simulink model "Model_TranslationEngine64"  (R2022b)
settings: Solver=FixedStepDiscrete  StartTime=0.0  StopTime=5  RelTol=1e-3  EnableMultiTasking=on
InitFcn:
  | % Initialize model
  | ModelSettings=BTConfig.GetModelSettings();
  | 
  | ModelSettings.Validate();
  | 
  | ModelInit;
  | 
  | 
  | % load library data
  | GainLibrary_data;
  | % Load saved values from partition process
  | CapturedConstMask.LoadMapFromFile(bdroot)
StartFcn:
  | % make sure all the simulated RTC requests are found
  | %RTC_SIM_OBJ.ValidateREQs();
undefined symbols (not defined in the file or in its folder): AA, BPLP, Column, NumHFRefBPF, NumHFRefLPF, NumMusicChannels, Row, VolumeMuteConfig
libraries: TuneVar x925, TOP x490, FeaturePath x111, CapturedConstLib x52
(part 10 of 34)

== system Model_TranslationEngine64/NEAR/Near1p1/VolumeMute/VolMuteCh4/Ann4NonEntGainCalc ==
  FeaturePath : FeaturePath/FeaturePath  FeatureName=Ann4NonEntGainCalc  IsGroup=off  GroupNumber=-1  IsModule=off  TriggerInit=[-350 -126 -235 -19]
      settings: SourceProductName=Bose Talaria
  TuneTOP : Subsystem  mask(Talaria Trivial Tune TOP){TriggerInit=[-380 277 -210 333], TopName=VncThresh, TuneName=VncThresh, DataTypeOut=single, MaskValue=Config.DefaultVncThresh, TunabilityNumber=1, MinValue=[], MaxValue=[], BankNumber=0, PreOverlay=false, PostOverlay=false, UseSameName=on}
      mask prompts: TriggerInit "Hidden: MoveFcn redraw"; TopName "Name:"; TuneName "Name of TuneVar:"; DataTypeOut "Data type:"; MaskValue "Default Value:"; TunabilityNumber "Tunability:"; MinValue "Min Value:"; MaxValue "Max Value:"; BankNumber "Target memory bank number:"; PreOverlay "Requires pre-overlay action:"; PostOverlay "Requires post-overlay action:"; UseSameName "Use same name for tune variable and TOP"
      mask help: The TuneTOP block encapsultes a Target Overlay Parameter, a Tune Variable, and a Trivial Translation between them.
      mask init:
      | [ok,activeTopPath,activeTunePath] = TuneTOP_Mask.Init(gcbh);
      settings: MoveFcn=TuneTOP_Mask.CB_TriggerInit(gcbh);
      mask Callback TriggerInit: TuneTOP_Mask.CB_TriggerInit(gcbh);
      mask TypeOptions TopName: TOP/TopName
      mask TypeOptions TuneName: Tune Variable/TuneName
      mask TypeOptions DataTypeOut: TOP/DataTypeOut
      mask TypeOptions MaskValue: Tune Variable/MaskValue
      mask TypeOptions TunabilityNumber: Tune Variable/TunabilityNumber
      mask Callback TunabilityNumber: TuneVarMask.CB_TunabilityNumber(gcbh);
      mask TypeOptions MinValue: Tune Variable/MinValue
      mask TypeOptions MaxValue: Tune Variable/MaxValue
      mask TypeOptions BankNumber: TOP/BankNumber
      mask TypeOptions PreOverlay: TOP/PreOverlay
      mask TypeOptions PostOverlay: TOP/PostOverlay
      mask Callback UseSameName: TuneTOP_Mask.CB_UseSameName(gcbh);
      mask DialogControl toolPanel Prompt: Tuning Tool Hints
      mask DialogControl DescriptionGroup Prompt: Description
      mask DialogControl EditDescription Prompt: Edit Description
      mask DialogControl EditDescription Callback: TuneTOP_Mask.CB_EditDescription(gcbh);
      mask DialogControl TunabilityText Prompt: Easy: Changes nearly every tuning.
      mask DialogControl AdvancedPanel Prompt: Advanced
      mask DialogControl ConvertToFullTranslation Prompt: Irreversible conversion to full translation
      mask DialogControl ConvertToFullTranslation Callback: TuneTOP_Mask.CB_ConvertToFullTranslation(gcbh);
      mask DialogControl ErrorContainer Prompt: Error Messages
      mask Display:
      | % retrieve icon definition
      | [path,w,h] = TuneTOP_Mask.Icon();
      | 
      | % retrieve the block's pixel size
      | pos = get(gcbh,'position');
      | bw = pos(3) - pos(1);
      | bh = pos(4) - pos(2);
      | 
      | % draw centered icon
      | xAdj = bw/2 - w/2 + 5;
      | yAdj = bh/2 - h/2 + 4;
      | for i=1:length(path)
      | 	patch(path(i).x+xAdj, path(i).y+yAdj, path(i).rgb);
      | end
      | 
      | % show the top name or an X
      | if (exist('ok','var') && ok)
      | 	text(bw*0.5, bh*0.2, activeTopPath, 'horizontalAlignment', 'center');
      | 	patch(0,0,[1 1 1]);
      | 	patch(bw,bh,[1 1 1]);
      | else
      | 	tx=bw*0.03;
      | 	ty=bh*0.03;
      | 	patch([0 tx bw bw-tx], [ty 0 bh-ty bh], [1 0 0]);
      | 	patch([0 bw-tx bw tx], [bh-ty 0 ty bh], [1 0 0]);
      | end
  TuneTOP1 : Subsystem  mask(Talaria Trivial Tune TOP){TriggerInit=[-380 347 -210 403], TopName=VncSlope, TuneName=VncSlope, DataTypeOut=single, MaskValue=Config.DefaultVncSlope, TunabilityNumber=1, MinValue=[], MaxValue=[], BankNumber=0, PreOverlay=false, PostOverlay=false, UseSameName=on}
      mask prompts: TriggerInit "Hidden: MoveFcn redraw"; TopName "Name:"; TuneName "Name of TuneVar:"; DataTypeOut "Data type:"; MaskValue "Default Value:"; TunabilityNumber "Tunability:"; MinValue "Min Value:"; MaxValue "Max Value:"; BankNumber "Target memory bank number:"; PreOverlay "Requires pre-overlay action:"; PostOverlay "Requires post-overlay action:"; UseSameName "Use same name for tune variable and TOP"
      mask help: The TuneTOP block encapsultes a Target Overlay Parameter, a Tune Variable, and a Trivial Translation between them.
      mask init:
      | [ok,activeTopPath,activeTunePath] = TuneTOP_Mask.Init(gcbh);
      settings: MoveFcn=TuneTOP_Mask.CB_TriggerInit(gcbh);
      mask Callback TriggerInit: TuneTOP_Mask.CB_TriggerInit(gcbh);
      mask TypeOptions TopName: TOP/TopName
      mask TypeOptions TuneName: Tune Variable/TuneName
      mask TypeOptions DataTypeOut: TOP/DataTypeOut
      mask TypeOptions MaskValue: Tune Variable/MaskValue
      mask TypeOptions TunabilityNumber: Tune Variable/TunabilityNumber
      mask Callback TunabilityNumber: TuneVarMask.CB_TunabilityNumber(gcbh);
      mask TypeOptions MinValue: Tune Variable/MinValue
      mask TypeOptions MaxValue: Tune Variable/MaxValue
      mask TypeOptions BankNumber: TOP/BankNumber
      mask TypeOptions PreOverlay: TOP/PreOverlay
      mask TypeOptions PostOverlay: TOP/PostOverlay
      mask Callback UseSameName: TuneTOP_Mask.CB_UseSameName(gcbh);
      mask DialogControl toolPanel Prompt: Tuning Tool Hints
      mask DialogControl DescriptionGroup Prompt: Description
      mask DialogControl EditDescription Prompt: Edit Description
      mask DialogControl EditDescription Callback: TuneTOP_Mask.CB_EditDescription(gcbh);
      mask DialogControl TunabilityText Prompt: Easy: Changes nearly every tuning.
      mask DialogControl AdvancedPanel Prompt: Advanced
      mask DialogControl ConvertToFullTranslation Prompt: Irreversible conversion to full translation
      mask DialogControl ConvertToFullTranslation Callback: TuneTOP_Mask.CB_ConvertToFullTranslation(gcbh);
      mask DialogControl ErrorContainer Prompt: Error Messages
      mask Display:
      | % retrieve icon definition
      | [path,w,h] = TuneTOP_Mask.Icon();
      | 
      | % retrieve the block's pixel size
      | pos = get(gcbh,'position');
      | bw = pos(3) - pos(1);
      | bh = pos(4) - pos(2);
      | 
      | % draw centered icon
      | xAdj = bw/2 - w/2 + 5;
      | yAdj = bh/2 - h/2 + 4;
      | for i=1:length(path)
      | 	patch(path(i).x+xAdj, path(i).y+yAdj, path(i).rgb);
      | end
      | 
      | % show the top name or an X
      | if (exist('ok','var') && ok)
      | 	text(bw*0.5, bh*0.2, activeTopPath, 'horizontalAlignment', 'center');
      | 	patch(0,0,[1 1 1]);
      | 	patch(bw,bh,[1 1 1]);
      | else
      | 	tx=bw*0.03;
      | 	ty=bh*0.03;
      | 	patch([0 tx bw bw-tx], [ty 0 bh-ty bh], [1 0 0]);
      | 	patch([0 bw-tx bw tx], [bh-ty 0 ty bh], [1 0 0]);
      | end
  TuneTOP2 : Subsystem  mask(Talaria Trivial Tune TOP){TriggerInit=[-380 427 -210 483], TopName=MaxBoost, TuneName=MaxBoost, DataTypeOut=single, MaskValue=Config.DefaultMaxBoost, TunabilityNumber=1, MinValue=[], MaxValue=[], BankNumber=0, PreOverlay=false, PostOverlay=false, UseSameName=on}
      mask prompts: TriggerInit "Hidden: MoveFcn redraw"; TopName "Name:"; TuneName "Name of TuneVar:"; DataTypeOut "Data type:"; MaskValue "Default Value:"; TunabilityNumber "Tunability:"; MinValue "Min Value:"; MaxValue "Max Value:"; BankNumber "Target memory bank number:"; PreOverlay "Requires pre-overlay action:"; PostOverlay "Requires post-overlay action:"; UseSameName "Use same name for tune variable and TOP"
      mask help: The TuneTOP block encapsultes a Target Overlay Parameter, a Tune Variable, and a Trivial Translation between them.
      mask init:
      | [ok,activeTopPath,activeTunePath] = TuneTOP_Mask.Init(gcbh);
      settings: MoveFcn=TuneTOP_Mask.CB_TriggerInit(gcbh);
      mask Callback TriggerInit: TuneTOP_Mask.CB_TriggerInit(gcbh);
      mask TypeOptions TopName: TOP/TopName
      mask TypeOptions TuneName: Tune Variable/TuneName
      mask TypeOptions DataTypeOut: TOP/DataTypeOut
      mask TypeOptions MaskValue: Tune Variable/MaskValue
      mask TypeOptions TunabilityNumber: Tune Variable/TunabilityNumber
      mask Callback TunabilityNumber: TuneVarMask.CB_TunabilityNumber(gcbh);
      mask TypeOptions MinValue: Tune Variable/MinValue
      mask TypeOptions MaxValue: Tune Variable/MaxValue
      mask TypeOptions BankNumber: TOP/BankNumber
      mask TypeOptions PreOverlay: TOP/PreOverlay
      mask TypeOptions PostOverlay: TOP/PostOverlay
      mask Callback UseSameName: TuneTOP_Mask.CB_UseSameName(gcbh);
      mask DialogControl toolPanel Prompt: Tuning Tool Hints
      mask DialogControl DescriptionGroup Prompt: Description
      mask DialogControl EditDescription Prompt: Edit Description
      mask DialogControl EditDescription Callback: TuneTOP_Mask.CB_EditDescription(gcbh);
      mask DialogControl TunabilityText Prompt: Easy: Changes nearly every tuning.
      mask DialogControl AdvancedPanel Prompt: Advanced
      mask DialogControl ConvertToFullTranslation Prompt: Irreversible conversion to full translation
      mask DialogControl ConvertToFullTranslation Callback: TuneTOP_Mask.CB_ConvertToFullTranslation(gcbh);
      mask DialogControl ErrorContainer Prompt: Error Messages
      mask Display:
      | % retrieve icon definition
      | [path,w,h] = TuneTOP_Mask.Icon();
      | 
      | % retrieve the block's pixel size
      | pos = get(gcbh,'position');
      | bw = pos(3) - pos(1);
      | bh = pos(4) - pos(2);
      | 
      | % draw centered icon
      | xAdj = bw/2 - w/2 + 5;
      | yAdj = bh/2 - h/2 + 4;
      | for i=1:length(path)
      | 	patch(path(i).x+xAdj, path(i).y+yAdj, path(i).rgb);
      | end
      | 
      | % show the top name or an X
      | if (exist('ok','var') && ok)
      | 	text(bw*0.5, bh*0.2, activeTopPath, 'horizontalAlignment', 'center');
      | 	patch(0,0,[1 1 1]);
      | 	patch(bw,bh,[1 1 1]);
      | else
      | 	tx=bw*0.03;
      | 	ty=bh*0.03;
      | 	patch([0 tx bw bw-tx], [ty 0 bh-ty bh], [1 0 0]);
      | 	patch([0 bw-tx bw tx], [bh-ty 0 ty bh], [1 0 0]);
      | end
  TuneTOP3 : Subsystem  mask(Talaria Trivial Tune TOP){TriggerInit=[-760 -98 -590 -42], TopName=NoiseOverRide, TuneName=NoiseOverRide, DataTypeOut=single, MaskValue=Config.DefaultNoiseOverride, TunabilityNumber=1, MinValue=[], MaxValue=[], BankNumber=0, PreOverlay=false, PostOverlay=false, UseSameName=on}
      mask prompts: TriggerInit "Hidden: MoveFcn redraw"; TopName "Name:"; TuneName "Name of TuneVar:"; DataTypeOut "Data type:"; MaskValue "Default Value:"; TunabilityNumber "Tunability:"; MinValue "Min Value:"; MaxValue "Max Value:"; BankNumber "Target memory bank number:"; PreOverlay "Requires pre-overlay action:"; PostOverlay "Requires post-overlay action:"; UseSameName "Use same name for tune variable and TOP"
      mask help: The TuneTOP block encapsultes a Target Overlay Parameter, a Tune Variable, and a Trivial Translation between them.
      mask init:
      | [ok,activeTopPath,activeTunePath] = TuneTOP_Mask.Init(gcbh);
      settings: MoveFcn=TuneTOP_Mask.CB_TriggerInit(gcbh);
      mask Callback TriggerInit: TuneTOP_Mask.CB_TriggerInit(gcbh);
      mask TypeOptions TopName: TOP/TopName
      mask TypeOptions TuneName: Tune Variable/TuneName
      mask TypeOptions DataTypeOut: TOP/DataTypeOut
      mask TypeOptions MaskValue: Tune Variable/MaskValue
      mask TypeOptions TunabilityNumber: Tune Variable/TunabilityNumber
      mask Callback TunabilityNumber: TuneVarMask.CB_TunabilityNumber(gcbh);
      mask TypeOptions MinValue: Tune Variable/MinValue
      mask TypeOptions MaxValue: Tune Variable/MaxValue
      mask TypeOptions BankNumber: TOP/BankNumber
      mask TypeOptions PreOverlay: TOP/PreOverlay
      mask TypeOptions PostOverlay: TOP/PostOverlay
      mask Callback UseSameName: TuneTOP_Mask.CB_UseSameName(gcbh);
      mask DialogControl toolPanel Prompt: Tuning Tool Hints
      mask DialogControl DescriptionGroup Prompt: Description
      mask DialogControl EditDescription Prompt: Edit Description
      mask DialogControl EditDescription Callback: TuneTOP_Mask.CB_EditDescription(gcbh);
      mask DialogControl TunabilityText Prompt: Easy: Changes nearly every tuning.
      mask DialogControl AdvancedPanel Prompt: Advanced
      mask DialogControl ConvertToFullTranslation Prompt: Irreversible conversion to full translation
      mask DialogControl ConvertToFullTranslation Callback: TuneTOP_Mask.CB_ConvertToFullTranslation(gcbh);
      mask DialogControl ErrorContainer Prompt: Error Messages
      mask Display:
      | % retrieve icon definition
      | [path,w,h] = TuneTOP_Mask.Icon();
      | 
      | % retrieve the block's pixel size
      | pos = get(gcbh,'position');
      | bw = pos(3) - pos(1);
      | bh = pos(4) - pos(2);
      | 
      | % draw centered icon
      | xAdj = bw/2 - w/2 + 5;
      | yAdj = bh/2 - h/2 + 4;
      | for i=1:length(path)
      | 	patch(path(i).x+xAdj, path(i).y+yAdj, path(i).rgb);
      | end
      | 
      | % show the top name or an X
      | if (exist('ok','var') && ok)
      | 	text(bw*0.5, bh*0.2, activeTopPath, 'horizontalAlignment', 'center');
      | 	patch(0,0,[1 1 1]);
      | 	patch(bw,bh,[1 1 1]);
      | else
      | 	tx=bw*0.03;
      | 	ty=bh*0.03;
      | 	patch([0 tx bw bw-tx], [ty 0 bh-ty bh], [1 0 0]);
      | 	patch([0 bw-tx bw tx], [bh-ty 0 ty bh], [1 0 0]);
      | end
  TuneTOP4 : Subsystem  mask(Talaria Trivial Tune TOP){TriggerInit=[-760 -18 -590 38], TopName=NoiseOverRideFlag, TuneName=NoiseOverRideFlag, DataTypeOut=single, MaskValue=Config.DefaultNoiseOverrideFlag, TunabilityNumber=1, MinValue=[], MaxValue=[], BankNumber=0, PreOverlay=false, PostOverlay=false, UseSameName=on}
      mask prompts: TriggerInit "Hidden: MoveFcn redraw"; TopName "Name:"; TuneName "Name of TuneVar:"; DataTypeOut "Data type:"; MaskValue "Default Value:"; TunabilityNumber "Tunability:"; MinValue "Min Value:"; MaxValue "Max Value:"; BankNumber "Target memory bank number:"; PreOverlay "Requires pre-overlay action:"; PostOverlay "Requires post-overlay action:"; UseSameName "Use same name for tune variable and TOP"
      mask help: The TuneTOP block encapsultes a Target Overlay Parameter, a Tune Variable, and a Trivial Translation between them.
      mask init:
      | [ok,activeTopPath,activeTunePath] = TuneTOP_Mask.Init(gcbh);
      settings: MoveFcn=TuneTOP_Mask.CB_TriggerInit(gcbh);
      mask Callback TriggerInit: TuneTOP_Mask.CB_TriggerInit(gcbh);
      mask TypeOptions TopName: TOP/TopName
      mask TypeOptions TuneName: Tune Variable/TuneName
      mask TypeOptions DataTypeOut: TOP/DataTypeOut
      mask TypeOptions MaskValue: Tune Variable/MaskValue
      mask TypeOptions TunabilityNumber: Tune Variable/TunabilityNumber
      mask Callback TunabilityNumber: TuneVarMask.CB_TunabilityNumber(gcbh);
      mask TypeOptions MinValue: Tune Variable/MinValue
      mask TypeOptions MaxValue: Tune Variable/MaxValue
      mask TypeOptions BankNumber: TOP/BankNumber
      mask TypeOptions PreOverlay: TOP/PreOverlay
      mask TypeOptions PostOverlay: TOP/PostOverlay
      mask Callback UseSameName: TuneTOP_Mask.CB_UseSameName(gcbh);
      mask DialogControl toolPanel Prompt: Tuning Tool Hints
      mask DialogControl DescriptionGroup Prompt: Description
      mask DialogControl EditDescription Prompt: Edit Description
      mask DialogControl EditDescription Callback: TuneTOP_Mask.CB_EditDescription(gcbh);
      mask DialogControl TunabilityText Prompt: Easy: Changes nearly every tuning.
      mask DialogControl AdvancedPanel Prompt: Advanced
      mask DialogControl ConvertToFullTranslation Prompt: Irreversible conversion to full translation
      mask DialogControl ConvertToFullTranslation Callback: TuneTOP_Mask.CB_ConvertToFullTranslation(gcbh);
      mask DialogControl ErrorContainer Prompt: Error Messages
      mask Display:
      | % retrieve icon definition
      | [path,w,h] = TuneTOP_Mask.Icon();
      | 
      | % retrieve the block's pixel size
      | pos = get(gcbh,'position');
      | bw = pos(3) - pos(1);
      | bh = pos(4) - pos(2);
      | 
      | % draw centered icon
      | xAdj = bw/2 - w/2 + 5;
      | yAdj = bh/2 - h/2 + 4;
      | for i=1:length(path)
      | 	patch(path(i).x+xAdj, path(i).y+yAdj, path(i).rgb);
      | end
      | 
      | % show the top name or an X
      | if (exist('ok','var') && ok)
      | 	text(bw*0.5, bh*0.2, activeTopPath, 'horizontalAlignment', 'center');
      | 	patch(0,0,[1 1 1]);
      | 	patch(bw,bh,[1 1 1]);
      | else
      | 	tx=bw*0.03;
      | 	ty=bh*0.03;
      | 	patch([0 tx bw bw-tx], [ty 0 bh-ty bh], [1 0 0]);
      | 	patch([0 bw-tx bw tx], [bh-ty 0 ty bh], [1 0 0]);
      | end
  TuneTOP5 : Subsystem  mask(Talaria Trivial Tune TOP){TriggerInit=[-760 157 -590 213], TopName=BoostOverRide, TuneName=BoostOverRide, DataTypeOut=single, MaskValue=Config.DefaultBoostOverride, TunabilityNumber=1, MinValue=[], MaxValue=[], BankNumber=0, PreOverlay=false, PostOverlay=false, UseSameName=on}
      mask prompts: TriggerInit "Hidden: MoveFcn redraw"; TopName "Name:"; TuneName "Name of TuneVar:"; DataTypeOut "Data type:"; MaskValue "Default Value:"; TunabilityNumber "Tunability:"; MinValue "Min Value:"; MaxValue "Max Value:"; BankNumber "Target memory bank number:"; PreOverlay "Requires pre-overlay action:"; PostOverlay "Requires post-overlay action:"; UseSameName "Use same name for tune variable and TOP"
      mask help: The TuneTOP block encapsultes a Target Overlay Parameter, a Tune Variable, and a Trivial Translation between them.
      mask init:
      | [ok,activeTopPath,activeTunePath] = TuneTOP_Mask.Init(gcbh);
      settings: MoveFcn=TuneTOP_Mask.CB_TriggerInit(gcbh);
      mask Callback TriggerInit: TuneTOP_Mask.CB_TriggerInit(gcbh);
      mask TypeOptions TopName: TOP/TopName
      mask TypeOptions TuneName: Tune Variable/TuneName
      mask TypeOptions DataTypeOut: TOP/DataTypeOut
      mask TypeOptions MaskValue: Tune Variable/MaskValue
      mask TypeOptions TunabilityNumber: Tune Variable/TunabilityNumber
      mask Callback TunabilityNumber: TuneVarMask.CB_TunabilityNumber(gcbh);
      mask TypeOptions MinValue: Tune Variable/MinValue
      mask TypeOptions MaxValue: Tune Variable/MaxValue
      mask TypeOptions BankNumber: TOP/BankNumber
      mask TypeOptions PreOverlay: TOP/PreOverlay
      mask TypeOptions PostOverlay: TOP/PostOverlay
      mask Callback UseSameName: TuneTOP_Mask.CB_UseSameName(gcbh);
      mask DialogControl toolPanel Prompt: Tuning Tool Hints
      mask DialogControl DescriptionGroup Prompt: Description
      mask DialogControl EditDescription Prompt: Edit Description
      mask DialogControl EditDescription Callback: TuneTOP_Mask.CB_EditDescription(gcbh);
      mask DialogControl TunabilityText Prompt: Easy: Changes nearly every tuning.
      mask DialogControl AdvancedPanel Prompt: Advanced
      mask DialogControl ConvertToFullTranslation Prompt: Irreversible conversion to full translation
      mask DialogControl ConvertToFullTranslation Callback: TuneTOP_Mask.CB_ConvertToFullTranslation(gcbh);
      mask DialogControl ErrorContainer Prompt: Error Messages
      mask Display:
      | % retrieve icon definition
      | [path,w,h] = TuneTOP_Mask.Icon();
      | 
      | % retrieve the block's pixel size
      | pos = get(gcbh,'position');
      | bw = pos(3) - pos(1);
      | bh = pos(4) - pos(2);
      | 
      | % draw centered icon
      | xAdj = bw/2 - w/2 + 5;
      | yAdj = bh/2 - h/2 + 4;
      | for i=1:length(path)
      | 	patch(path(i).x+xAdj, path(i).y+yAdj, path(i).rgb);
      | end
      | 
      | % show the top name or an X
      | if (exist('ok','var') && ok)
      | 	text(bw*0.5, bh*0.2, activeTopPath, 'horizontalAlignment', 'center');
      | 	patch(0,0,[1 1 1]);
      | 	patch(bw,bh,[1 1 1]);
      | else
      | 	tx=bw*0.03;
      | 	ty=bh*0.03;
      | 	patch([0 tx bw bw-tx], [ty 0 bh-ty bh], [1 0 0]);
      | 	patch([0 bw-tx bw tx], [bh-ty 0 ty bh], [1 0 0]);
      | end
  TuneTOP6 : Subsystem  mask(Talaria Trivial Tune TOP){TriggerInit=[-760 232 -590 288], TopName=BoostOverRideFlag, TuneName=BoostOverRideFlag, DataTypeOut=single, MaskValue=Config.DefaultBoostOverrideFlag, TunabilityNumber=1, MinValue=[], MaxValue=[], BankNumber=0, PreOverlay=false, PostOverlay=false, UseSameName=on}
      mask prompts: TriggerInit "Hidden: MoveFcn redraw"; TopName "Name:"; TuneName "Name of TuneVar:"; DataTypeOut "Data type:"; MaskValue "Default Value:"; TunabilityNumber "Tunability:"; MinValue "Min Value:"; MaxValue "Max Value:"; BankNumber "Target memory bank number:"; PreOverlay "Requires pre-overlay action:"; PostOverlay "Requires post-overlay action:"; UseSameName "Use same name for tune variable and TOP"
      mask help: The TuneTOP block encapsultes a Target Overlay Parameter, a Tune Variable, and a Trivial Translation between them.
      mask init:
      | [ok,activeTopPath,activeTunePath] = TuneTOP_Mask.Init(gcbh);
      settings: MoveFcn=TuneTOP_Mask.CB_TriggerInit(gcbh);
      mask Callback TriggerInit: TuneTOP_Mask.CB_TriggerInit(gcbh);
      mask TypeOptions TopName: TOP/TopName
      mask TypeOptions TuneName: Tune Variable/TuneName
      mask TypeOptions DataTypeOut: TOP/DataTypeOut
      mask TypeOptions MaskValue: Tune Variable/MaskValue
      mask TypeOptions TunabilityNumber: Tune Variable/TunabilityNumber
      mask Callback TunabilityNumber: TuneVarMask.CB_TunabilityNumber(gcbh);
      mask TypeOptions MinValue: Tune Variable/MinValue
      mask TypeOptions MaxValue: Tune Variable/MaxValue
      mask TypeOptions BankNumber: TOP/BankNumber
      mask TypeOptions PreOverlay: TOP/PreOverlay
      mask TypeOptions PostOverlay: TOP/PostOverlay
      mask Callback UseSameName: TuneTOP_Mask.CB_UseSameName(gcbh);
      mask DialogControl toolPanel Prompt: Tuning Tool Hints
      mask DialogControl DescriptionGroup Prompt: Description
      mask DialogControl EditDescription Prompt: Edit Description
      mask DialogControl EditDescription Callback: TuneTOP_Mask.CB_EditDescription(gcbh);
      mask DialogControl TunabilityText Prompt: Easy: Changes nearly every tuning.
      mask DialogControl AdvancedPanel Prompt: Advanced
      mask DialogControl ConvertToFullTranslation Prompt: Irreversible conversion to full translation
      mask DialogControl ConvertToFullTranslation Callback: TuneTOP_Mask.CB_ConvertToFullTranslation(gcbh);
      mask DialogControl ErrorContainer Prompt: Error Messages
      mask Display:
      | % retrieve icon definition
      | [path,w,h] = TuneTOP_Mask.Icon();
      | 
      | % retrieve the block's pixel size
      | pos = get(gcbh,'position');
      | bw = pos(3) - pos(1);
      | bh = pos(4) - pos(2);
      | 
      | % draw centered icon
      | xAdj = bw/2 - w/2 + 5;
      | yAdj = bh/2 - h/2 + 4;
      | for i=1:length(path)
      | 	patch(path(i).x+xAdj, path(i).y+yAdj, path(i).rgb);
      | end
      | 
      | % show the top name or an X
      | if (exist('ok','var') && ok)
      | 	text(bw*0.5, bh*0.2, activeTopPath, 'horizontalAlignment', 'center');
      | 	patch(0,0,[1 1 1]);
      | 	patch(bw,bh,[1 1 1]);
      | else
      | 	tx=bw*0.03;
      | 	ty=bh*0.03;
      | 	patch([0 tx bw bw-tx], [ty 0 bh-ty bh], [1 0 0]);
      | 	patch([0 bw-tx bw tx], [bh-ty 0 ty bh], [1 0 0]);
      | end
  TuneTOP7 : Subsystem  mask(Talaria Trivial Tune TOP){TriggerInit=[-1110 322 -940 378], TopName=VncEnableTuneVar, TuneName=VncEnableTuneVar, DataTypeOut=single, MaskValue=Config.DefaultVncEnable, TunabilityNumber=1, MinValue=[], MaxValue=[], BankNumber=0, PreOverlay=false, PostOverlay=false, UseSameName=on}
      mask prompts: TriggerInit "Hidden: MoveFcn redraw"; TopName "Name:"; TuneName "Name of TuneVar:"; DataTypeOut "Data type:"; MaskValue "Default Value:"; TunabilityNumber "Tunability:"; MinValue "Min Value:"; MaxValue "Max Value:"; BankNumber "Target memory bank number:"; PreOverlay "Requires pre-overlay action:"; PostOverlay "Requires post-overlay action:"; UseSameName "Use same name for tune variable and TOP"
      mask help: The TuneTOP block encapsultes a Target Overlay Parameter, a Tune Variable, and a Trivial Translation between them.
      mask init:
      | [ok,activeTopPath,activeTunePath] = TuneTOP_Mask.Init(gcbh);
      settings: MoveFcn=TuneTOP_Mask.CB_TriggerInit(gcbh);
      mask Callback TriggerInit: TuneTOP_Mask.CB_TriggerInit(gcbh);
      mask TypeOptions TopName: TOP/TopName
      mask TypeOptions TuneName: Tune Variable/TuneName
      mask TypeOptions DataTypeOut: TOP/DataTypeOut
      mask TypeOptions MaskValue: Tune Variable/MaskValue
      mask TypeOptions TunabilityNumber: Tune Variable/TunabilityNumber
      mask Callback TunabilityNumber: TuneVarMask.CB_TunabilityNumber(gcbh);
      mask TypeOptions MinValue: Tune Variable/MinValue
      mask TypeOptions MaxValue: Tune Variable/MaxValue
      mask TypeOptions BankNumber: TOP/BankNumber
      mask TypeOptions PreOverlay: TOP/PreOverlay
      mask TypeOptions PostOverlay: TOP/PostOverlay
      mask Callback UseSameName: TuneTOP_Mask.CB_UseSameName(gcbh);
      mask DialogControl toolPanel Prompt: Tuning Tool Hints
      mask DialogControl DescriptionGroup Prompt: Description
      mask DialogControl EditDescription Prompt: Edit Description
      mask DialogControl EditDescription Callback: TuneTOP_Mask.CB_EditDescription(gcbh);
      mask DialogControl TunabilityText Prompt: Easy: Changes nearly every tuning.
      mask DialogControl AdvancedPanel Prompt: Advanced
      mask DialogControl ConvertToFullTranslation Prompt: Irreversible conversion to full translation
      mask DialogControl ConvertToFullTranslation Callback: TuneTOP_Mask.CB_ConvertToFullTranslation(gcbh);
      mask DialogControl ErrorContainer Prompt: Error Messages
      mask Display:
      | % retrieve icon definition
      | [path,w,h] = TuneTOP_Mask.Icon();
      | 
      | % retrieve the block's pixel size
      | pos = get(gcbh,'position');
      | bw = pos(3) - pos(1);
      | bh = pos(4) - pos(2);
      | 
      | % draw centered icon
      | xAdj = bw/2 - w/2 + 5;
      | yAdj = bh/2 - h/2 + 4;
      | for i=1:length(path)
      | 	patch(path(i).x+xAdj, path(i).y+yAdj, path(i).rgb);
      | end
      | 
      | % show the top name or an X
      | if (exist('ok','var') && ok)
      | 	text(bw*0.5, bh*0.2, activeTopPath, 'horizontalAlignment', 'center');
      | 	patch(0,0,[1 1 1]);
      | 	patch(bw,bh,[1 1 1]);
      | else
      | 	tx=bw*0.03;
      | 	ty=bh*0.03;
      | 	patch([0 tx bw bw-tx], [ty 0 bh-ty bh], [1 0 0]);
      | 	patch([0 bw-tx bw tx], [bh-ty 0 ty bh], [1 0 0]);
      | end
  TuneTOP8 : Subsystem
  vncSignal : Subsystem

== system Model_TranslationEngine64/NEAR/Near1p1/VolumeMute/VolMuteCh4/Ann4NonEntVncApplied ==
  FeaturePath : FeaturePath/FeaturePath  FeatureName=Ann4NonEntVncApplied  IsGroup=off  GroupNumber=-1  IsModule=off  TriggerInit=[500 179 625 271]
      settings: SourceProductName=Bose Talaria
  nonentVNCApplied_subsystem : Subsystem

== system Model_TranslationEngine64/NEAR/Near1p1/VolumeMute/VolMuteCh4/Mute ==
  MuteControl : Subsystem  mask(Blocklib MuteControl){Config=Config, FeatureName=Ann4Mute}
      mask prompts: Config "MuteControlConfig"; FeatureName "Mask feature name:"
      mask help: This component is to be used in conjunction with 1 or more instances of the MuteRamper block. There is no mask for this component. It provides the control layer for Mute processing via an RTC and tune variable, muteControlRampTime.
      mask init: same as Model_TranslationEngine64/PostProcess/PostProcess/Mute/Mute/MuteControl
      mask Help: If this control block is being used in a "multi-instance" manner, i.e. it is contorlling two or more MuteRamper blocks, there is an additional step that must be done. The developer must add a function-triggered subsytem containing an AND logic gate, which will combine the notification completion signals of the multiple ramper instances. The output of this subsytem must then feed the NTF_done input of the MuteControl block.
      mask Callback Config: BTConfig.CallbackHideIfPresent(gcbh,{'FeatureName'});
      mask TypeOptions FeatureName: FeaturePath/FeatureName

== system Model_TranslationEngine64/NEAR/Near1p1/VolumeMute/VolMuteCh4/Volume ==
  FeaturePath : FeaturePath/FeaturePath  FeatureName=Ann4Volume  IsGroup=off  GroupNumber=-1  IsModule=off  TriggerInit=[-260 -306 -145 -199]
      settings: SourceProductName=Bose Talaria
  TOP_GainDB : TOP/TOP  TriggerInit=[380 -243 530 -187]  TopName=Table_dB  DataTypeOut=Inherit: Same as input  BankNumber=Config.BankNumber  PreOverlay=false  PostOverlay=false  Role=Automatic
      settings: SourceProductName=Bose Talaria
  TOP_Index : TOP/TOP  TriggerInit=[380 -313 530 -257]  TopName=Table_Idx  DataTypeOut=Inherit: Same as input  BankNumber=Config.BankNumber  PreOverlay=false  PostOverlay=false  Role=Automatic
      settings: SourceProductName=Bose Talaria
  TranslateTrigger1 : TuneVar/TranslateTrigger  TriggerInit=[211 -395 249 -345]
      settings: SourceProductName=Bose Talaria
  TuneVarRampRate : Subsystem  mask(Talaria Trivial Tune TOP){TriggerInit=[-95 52 75 108], TopName=RampRate, TuneName=RampRate, DataTypeOut=single, MaskValue=100, TunabilityNumber=2, MinValue=5, MaxValue=50000, BankNumber=0, PreOverlay=false, PostOverlay=false, UseSameName=on}
      mask prompts: TriggerInit "Hidden: MoveFcn redraw"; TopName "Name:"; TuneName "Name of TuneVar:"; DataTypeOut "Data type:"; MaskValue "Default Value:"; TunabilityNumber "Tunability:"; MinValue "Min Value:"; MaxValue "Max Value:"; BankNumber "Target memory bank number:"; PreOverlay "Requires pre-overlay action:"; PostOverlay "Requires post-overlay action:"; UseSameName "Use same name for tune variable and TOP"
      mask help: The TuneTOP block encapsultes a Target Overlay Parameter, a Tune Variable, and a Trivial Translation between them.
      mask init:
      | [ok,activeTopPath,activeTunePath] = TuneTOP_Mask.Init(gcbh);
      settings: MoveFcn=TuneTOP_Mask.CB_TriggerInit(gcbh);
      mask Callback TriggerInit: TuneTOP_Mask.CB_TriggerInit(gcbh);
      mask TypeOptions TopName: TOP/TopName
      mask TypeOptions TuneName: Tune Variable/TuneName
      mask TypeOptions DataTypeOut: TOP/DataTypeOut
      mask TypeOptions MaskValue: Tune Variable/MaskValue
      mask TypeOptions TunabilityNumber: Tune Variable/TunabilityNumber
      mask Callback TunabilityNumber: TuneVarMask.CB_TunabilityNumber(gcbh);
      mask TypeOptions MinValue: Tune Variable/MinValue
      mask TypeOptions MaxValue: Tune Variable/MaxValue
      mask TypeOptions BankNumber: TOP/BankNumber
      mask TypeOptions PreOverlay: TOP/PreOverlay
      mask TypeOptions PostOverlay: TOP/PostOverlay
      mask Callback UseSameName: TuneTOP_Mask.CB_UseSameName(gcbh);
      mask DialogControl toolPanel Prompt: Tuning Tool Hints
      mask DialogControl DescriptionGroup Prompt: Description
      mask DialogControl EditDescription Prompt: Edit Description
      mask DialogControl EditDescription Callback: TuneTOP_Mask.CB_EditDescription(gcbh);
      mask DialogControl TunabilityText Prompt: Easy: Changes nearly every tuning.
      mask DialogControl AdvancedPanel Prompt: Advanced
      mask DialogControl ConvertToFullTranslation Prompt: Irreversible conversion to full translation
      mask DialogControl ConvertToFullTranslation Callback: TuneTOP_Mask.CB_ConvertToFullTranslation(gcbh);
      mask DialogControl ErrorContainer Prompt: Error Messages
      mask Display:
      | % retrieve icon definition
      | [path,w,h] = TuneTOP_Mask.Icon();
      | 
      | % retrieve the block's pixel size
      | pos = get(gcbh,'position');
      | bw = pos(3) - pos(1);
      | bh = pos(4) - pos(2);
      | 
      | % draw centered icon
      | xAdj = bw/2 - w/2 + 5;
      | yAdj = bh/2 - h/2 + 4;
      | for i=1:length(path)
      | 	patch(path(i).x+xAdj, path(i).y+yAdj, path(i).rgb);
      | end
      | 
      | % show the top name or an X
      | if (exist('ok','var') && ok)
      | 	text(bw*0.5, bh*0.2, activeTopPath, 'horizontalAlignment', 'center');
      | 	patch(0,0,[1 1 1]);
      | 	patch(bw,bh,[1 1 1]);
      | else
      | 	tx=bw*0.03;
      | 	ty=bh*0.03;
      | 	patch([0 tx bw bw-tx], [ty 0 bh-ty bh], [1 0 0]);
      | 	patch([0 bw-tx bw tx], [bh-ty 0 ty bh], [1 0 0]);
      | end
  TuneVarRampTime : Subsystem  mask(Talaria Trivial Tune TOP){TriggerInit=[-95 -28 75 28], TopName=RampTime, TuneName=RampTime, DataTypeOut=single, MaskValue=100, TunabilityNumber=1, MinValue=[], MaxValue=[], BankNumber=0, PreOverlay=false, PostOverlay=false, UseSameName=on}
      mask prompts: TriggerInit "Hidden: MoveFcn redraw"; TopName "Name:"; TuneName "Name of TuneVar:"; DataTypeOut "Data type:"; MaskValue "Default Value:"; TunabilityNumber "Tunability:"; MinValue "Min Value:"; MaxValue "Max Value:"; BankNumber "Target memory bank number:"; PreOverlay "Requires pre-overlay action:"; PostOverlay "Requires post-overlay action:"; UseSameName "Use same name for tune variable and TOP"
      mask help: The TuneTOP block encapsultes a Target Overlay Parameter, a Tune Variable, and a Trivial Translation between them.
      mask init:
      | [ok,activeTopPath,activeTunePath] = TuneTOP_Mask.Init(gcbh);
      settings: MoveFcn=TuneTOP_Mask.CB_TriggerInit(gcbh);
      mask Callback TriggerInit: TuneTOP_Mask.CB_TriggerInit(gcbh);
      mask TypeOptions TopName: TOP/TopName
      mask TypeOptions TuneName: Tune Variable/TuneName
      mask TypeOptions DataTypeOut: TOP/DataTypeOut
      mask TypeOptions MaskValue: Tune Variable/MaskValue
      mask TypeOptions TunabilityNumber: Tune Variable/TunabilityNumber
      mask Callback TunabilityNumber: TuneVarMask.CB_TunabilityNumber(gcbh);
      mask TypeOptions MinValue: Tune Variable/MinValue
      mask TypeOptions MaxValue: Tune Variable/MaxValue
      mask TypeOptions BankNumber: TOP/BankNumber
      mask TypeOptions PreOverlay: TOP/PreOverlay
      mask TypeOptions PostOverlay: TOP/PostOverlay
      mask Callback UseSameName: TuneTOP_Mask.CB_UseSameName(gcbh);
      mask DialogControl toolPanel Prompt: Tuning Tool Hints
      mask DialogControl DescriptionGroup Prompt: Description
      mask DialogControl EditDescription Prompt: Edit Description
      mask DialogControl EditDescription Callback: TuneTOP_Mask.CB_EditDescription(gcbh);
      mask DialogControl TunabilityText Prompt: Easy: Changes nearly every tuning.
      mask DialogControl AdvancedPanel Prompt: Advanced
      mask DialogControl ConvertToFullTranslation Prompt: Irreversible conversion to full translation
      mask DialogControl ConvertToFullTranslation Callback: TuneTOP_Mask.CB_ConvertToFullTranslation(gcbh);
      mask DialogControl ErrorContainer Prompt: Error Messages
      mask Display:
      | % retrieve icon definition
      | [path,w,h] = TuneTOP_Mask.Icon();
      | 
      | % retrieve the block's pixel size
      | pos = get(gcbh,'position');
      | bw = pos(3) - pos(1);
      | bh = pos(4) - pos(2);
      | 
      | % draw centered icon
      | xAdj = bw/2 - w/2 + 5;
      | yAdj = bh/2 - h/2 + 4;
      | for i=1:length(path)
      | 	patch(path(i).x+xAdj, path(i).y+yAdj, path(i).rgb);
      | end
      | 
      | % show the top name or an X
      | if (exist('ok','var') && ok)
      | 	text(bw*0.5, bh*0.2, activeTopPath, 'horizontalAlignment', 'center');
      | 	patch(0,0,[1 1 1]);
      | 	patch(bw,bh,[1 1 1]);
      | else
      | 	tx=bw*0.03;
      | 	ty=bh*0.03;
      | 	patch([0 tx bw bw-tx], [ty 0 bh-ty bh], [1 0 0]);
      | 	patch([0 bw-tx bw tx], [bh-ty 0 ty bh], [1 0 0]);
      | end
  TuneVarVolumeTable : TuneVar/TuneVar  Description=|  TuneName=Table  SpecifyMaxSize=on  VariableDim=1 (Row)  MaxSize=[16 2]  TunabilityNumber=2  MinValue=[0;-100]  MaxValue=[1;0]  TriggerInit=[-95 -275 75 -225]  MaskValue=[[1 32 64 96 128 160 192 224] / 255; [-126.5 -100 -90 -40 -30 -20 -10 0.0]]'
      | <HTML>Gain table maps index to gain.
      | The index values are <FONT color="red">normalized</Font> floats between 0 and 1 while the gains are in dB (i.e. 0 implies no attenuation).
      | </html>
      settings: SourceProductName=Bose Talaria
  volume table translation : MATLAB Function  TreatAsAtomicUnit=on
  wires:
  TranslateTrigger1/1 -> volume table translation/Trigger
  TuneVarVolumeTable/1 -> volume table translation/1(VolumeTable)  "Table"
  volume table translation/1(Table_Idx) -> TOP_Index/1
  volume table translation/2(Table_dB) -> TOP_GainDB/1

== system Model_TranslationEngine64/PostProcess/PostProcess/Mute/Mute/MuteControl ==
  FeaturePath : FeaturePath/FeaturePath  FeatureName=Mute  IsGroup=off  GroupNumber=-1  IsModule=off  TriggerInit=[180 39 295 146]
      settings: SourceProductName=Bose Talaria
  TuneVarRampTime : Subsystem  Description=|  mask(Talaria Trivial Tune TOP){TriggerInit=[295 232 465 288], TopName=RampTime, TuneName=RampTime, DataTypeOut=single, MaskValue=Config.DefaultRampTimeMsec, TunabilityNumber=1, MinValue=1, MaxValue=100000, BankNumber=0, PreOverlay=false, PostOverlay=false, UseSameName=on}
      | Specifies the default value of ramp time for the Mute or Unmute operation.
      | Used only when the RTC message does not contain either ramp rate or ramp time.
      mask prompts: TriggerInit "Hidden: MoveFcn redraw"; TopName "Name:"; TuneName "Name of TuneVar:"; DataTypeOut "Data type:"; MaskValue "Default Value:"; TunabilityNumber "Tunability:"; MinValue "Min Value:"; MaxValue "Max Value:"; BankNumber "Target memory bank number:"; PreOverlay "Requires pre-overlay action:"; PostOverlay "Requires post-overlay action:"; UseSameName "Use same name for tune variable and TOP"
      mask help: The TuneTOP block encapsultes a Target Overlay Parameter, a Tune Variable, and a Trivial Translation between them.
      mask init:
      | [ok,activeTopPath,activeTunePath] = TuneTOP_Mask.Init(gcbh);
      settings: MoveFcn=TuneTOP_Mask.CB_TriggerInit(gcbh);
      mask Callback TriggerInit: TuneTOP_Mask.CB_TriggerInit(gcbh);
      mask TypeOptions TopName: TOP/TopName
      mask TypeOptions TuneName: Tune Variable/TuneName
      mask TypeOptions DataTypeOut: TOP/DataTypeOut
      mask TypeOptions MaskValue: Tune Variable/MaskValue
      mask TypeOptions TunabilityNumber: Tune Variable/TunabilityNumber
      mask Callback TunabilityNumber: TuneVarMask.CB_TunabilityNumber(gcbh);
      mask TypeOptions MinValue: Tune Variable/MinValue
      mask TypeOptions MaxValue: Tune Variable/MaxValue
      mask TypeOptions BankNumber: TOP/BankNumber
      mask TypeOptions PreOverlay: TOP/PreOverlay
      mask TypeOptions PostOverlay: TOP/PostOverlay
      mask Callback UseSameName: TuneTOP_Mask.CB_UseSameName(gcbh);
      mask DialogControl toolPanel Prompt: Tuning Tool Hints
      mask DialogControl DescriptionGroup Prompt: Description
      mask DialogControl EditDescription Prompt: Edit Description
      mask DialogControl EditDescription Callback: TuneTOP_Mask.CB_EditDescription(gcbh);
      mask DialogControl TunabilityText Prompt: Easy: Changes nearly every tuning.
      mask DialogControl AdvancedPanel Prompt: Advanced
      mask DialogControl ConvertToFullTranslation Prompt: Irreversible conversion to full translation
      mask DialogControl ConvertToFullTranslation Callback: TuneTOP_Mask.CB_ConvertToFullTranslation(gcbh);
      mask DialogControl ErrorContainer Prompt: Error Messages
      mask Display:
      | % retrieve icon definition
      | [path,w,h] = TuneTOP_Mask.Icon();
      | 
      | % retrieve the block's pixel size
      | pos = get(gcbh,'position');
      | bw = pos(3) - pos(1);
      | bh = pos(4) - pos(2);
      | 
      | % draw centered icon
      | xAdj = bw/2 - w/2 + 5;
      | yAdj = bh/2 - h/2 + 4;
      | for i=1:length(path)
      | 	patch(path(i).x+xAdj, path(i).y+yAdj, path(i).rgb);
      | end
      | 
      | % show the top name or an X
      | if (exist('ok','var') && ok)
      | 	text(bw*0.5, bh*0.2, activeTopPath, 'horizontalAlignment', 'center');
      | 	patch(0,0,[1 1 1]);
      | 	patch(bw,bh,[1 1 1]);
      | else
      | 	tx=bw*0.03;
      | 	ty=bh*0.03;
      | 	patch([0 tx bw bw-tx], [ty 0 bh-ty bh], [1 0 0]);
      | 	patch([0 bw-tx bw tx], [bh-ty 0 ty bh], [1 0 0]);
      | end

== system Model_TranslationEngine64/TestRouter/ASDRouter/InnerLink/AuxChannel_with_MATLAB_function/TuneTOP_enable_aux_flag ==
  TOP : TOP/TOP  TriggerInit=[440 20 585 80]  TopName=EnableAux  DataTypeOut=int32  BankNumber=BankNumber  PreOverlay=PreOverlay  PostOverlay=PostOverlay  Role=Automatic
      settings: SourceProductName=Bose Talaria
  TrivialTranslation : TuneVar/TrivialTranslation  TriggerInit=[300 28 350 72]
      settings: SourceProductName=Bose Talaria
  Tune Variable : TuneVar/TuneVar  TuneName=EnableAux  SpecifyMaxSize=off  VariableDim=1 (Row)  MaxSize=[1 1]  TunabilityNumber=1  MinValue=MinValue  MaxValue=MaxValue  TriggerInit=[20 25 190 75]  MaskValue=MaskValue
      settings: SourceProductName=Bose Talaria
  wires:
  Tune Variable/1 -> TrivialTranslation/1  "EnableAux"
  TrivialTranslation/1 -> TOP/1

== system Model_TranslationEngine64/TestRouter/ASDRouter/InnerLink/MainChannelSystem/TuneTOP_pmain_select ==
  TOP : TOP/TOP  TriggerInit=[440 20 585 80]  TopName=MainSelect  DataTypeOut=int32  BankNumber=BankNumber  PreOverlay=PreOverlay  PostOverlay=PostOverlay  Role=Automatic
      settings: SourceProductName=Bose Talaria
  TrivialTranslation : TuneVar/TrivialTranslation  TriggerInit=[300 28 350 72]
      settings: SourceProductName=Bose Talaria
  Tune Variable : TuneVar/TuneVar  TuneName=MainSelect  SpecifyMaxSize=off  VariableDim=1 (Row)  MaxSize=[1 1]  TunabilityNumber=1  MinValue=MinValue  MaxValue=MaxValue  TriggerInit=[20 25 190 75]  MaskValue=MaskValue
      settings: SourceProductName=Bose Talaria
  wires:
  Tune Variable/1 -> TrivialTranslation/1  "MainSelect"
  TrivialTranslation/1 -> TOP/1

== system Model_TranslationEngine64/ModelPreAmp/DecRate/AudioPilot35/Audiopilot_3_5/ConfigurationRtcInputs/AudiopilotTwoDowngrade ==
  TOP : TOP/TOP  TriggerInit=[440 20 585 80]  TopName=TwoDowngrade  DataTypeOut=uint32  BankNumber=BankNumber  PreOverlay=PreOverlay  PostOverlay=PostOverlay  Role=Automatic
      settings: SourceProductName=Bose Talaria
  TrivialTranslation : TuneVar/TrivialTranslation  TriggerInit=[300 28 350 72]
      settings: SourceProductName=Bose Talaria
  Tune Variable : TuneVar/TuneVar  TuneName=TwoDowngrade  SpecifyMaxSize=off  VariableDim=1 (Row)  MaxSize=[1 1]  TunabilityNumber=1  MinValue=MinValue  MaxValue=MaxValue  TriggerInit=[20 25 190 75]  MaskValue=MaskValue
      settings: SourceProductName=Bose Talaria
  wires:
  TrivialTranslation/1 -> TOP/1
  Tune Variable/1 -> TrivialTranslation/1  "TwoDowngrade"

== system Model_TranslationEngine64/ModelPreAmp/DecRate/AudioPilot35/Audiopilot_3_5/ConfigurationRtcInputs/Hvac ==
  table : Subsystem

== system Model_TranslationEngine64/ModelPreAmp/DecRate/AudioPilot35/Audiopilot_3_5/GainApplication/Compensation ==
  AntizipperRampLpf : Subsystem
  BassBpf : Subsystem
  MidrangeLpf : Subsystem
  MidrangeLpfAlignDelay : Subsystem
